simulink model "untitled"  (R2018a)
settings: Solver=ode4  StartTime=0.0  StopTime=40  FixedStep=0.1  RelTol=1e-3
values from neighbouring files (symbols this model uses):
  K = 1.35*(1+0.18*tau/(1-tau))/alfa    [PIDtun_CC.m]
  L = coor1(1)    [h2KTL.m]
  T = interp1(he(Lapparent+1:n,2), he(Lapparent+1:n,1),0.63*Ko)-coor1(1)    [h2KTL.m]
libraries: cstblocks x1
settings Model: Creator=spectra  LastModifiedBy=spectra

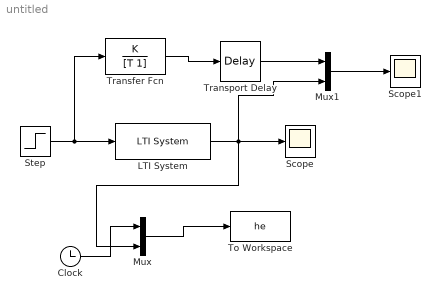
== system untitled ==
  Clock : Clock
  LTI System : cstblocks/LTI System  sys=tf(1,conv([2 1],[5 1]))  IC=[]
  Mux : Mux  Inputs=2
  Mux1 : Mux  Inputs=2
  Scope : Scope
  Scope1 : Scope
  Step : Step  Time=0  SampleTime=0
  To Workspace : ToWorkspace  VariableName=he  SaveFormat=Timeseries  SampleTime=-1
  Transfer Fcn : TransferFcn  Numerator=K  Denominator=[T 1]
  Transport Delay : TransportDelay  DelayTime=L
  wires:
  LTI System/1 -> Mux1/2, Mux/2, Scope/1
  Step/1 -> Transfer Fcn/1, LTI System/1
  Mux/1 -> To Workspace/1
  Clock/1 -> Mux/1
  Transfer Fcn/1 -> Transport Delay/1
  Transport Delay/1 -> Mux1/1
  Mux1/1 -> Scope1/1
